simulink model "Integration2022b_May06"  (R2022b)
settings: Solver=FixedStepAuto  StartTime=0.0  StopTime=inf  RelTol=1e-3
model workspace (MAT data in the model file):
  L = 4.165
  SL_ROS_VariableLengthArrays_MaxSizes : object (value not decoded)
  finalint = 0
  firstWarning = 1
  originalScenarioChecksum = '114339432DE22364D47BB28FC96DC10C'
values from neighbouring files (symbols this model uses):
  D = cross(B-A,C-A)    [HelperCalculateEgoRefPathInfo.m]
  data =     [Part_of_MCity.mat]    (also in curvedroad_Bhanu.mat; plotWPScript.m = [data, [out.x.Data(:, :, i); out.y.Data(:, :, i)]])
  x = [Vertices(Na,1) Vertices(:,1) Vertices(Nb,1)]    [HelperCalculateEgoRefPathInfo.m]    (also in HelperConvertDSPoseToSim3D.m = actor(1).Position(1); xpts.mat = [-29.9023190589 -34.2715935353 -19.4160603154 -19.4160603154)
  y = [Vertices(Na,2) Vertices(:,2) Vertices(Nb,2)]    [HelperCalculateEgoRefPathInfo.m]    (also in HelperConvertDSPoseToSim3D.m = actor(1).Position(2); VehicleOutputFcn.m = [x(1);x(2); x(3); x(4); x(5);x(6)]; ypts.mat = [-62.3254015256 -62.9079714558 -51.8391427821 -48.6350081661)
  z = zeros(1, length(interpX))    [HelperCalculateEgoRefPathInfo.m]
undefined symbols (not defined in the file or in its folder): MinVelocity, WB
libraries: ros2lib x13, mpcsigdimcheck_private x10, robotalgslib x1, mpclib x1, drivingvehiclecontroller x1, slpidlib x1
(part 2 of 5)

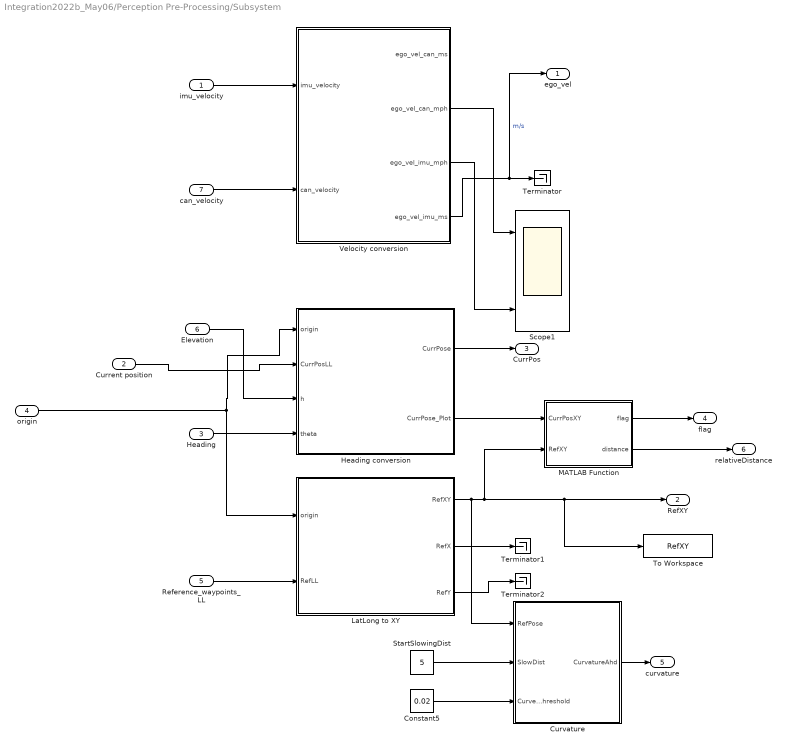
== system Integration2022b_May06/Perception Pre-Processing/Subsystem ==
  imu_velocity : Inport
  Current position : Inport  Port=2
  Heading : Inport  Port=3
  origin : Inport  Port=4
  Reference_waypoints_LL : Inport  Port=5
  Elevation : Inport  Port=6
  can_velocity : Inport  Port=7
  Constant5 : Constant  Value=0.02
  Curvature : MATLAB Function  TreatAsAtomicUnit=on
  Heading conversion : MATLAB Function  TreatAsAtomicUnit=on
  LatLong to XY : MATLAB Function  TreatAsAtomicUnit=on
  MATLAB Function : MATLAB Function  TreatAsAtomicUnit=on
  Scope1 : Scope  NumInputPorts=3
  StartSlowingDist : Constant  Value=5
  Terminator : Terminator
  Terminator1 : Terminator
  Terminator2 : Terminator
  To Workspace : ToWorkspace  VariableName=RefXY  SampleTime=-1
      settings: Save2DSignal=2-D array (concatenate along first dimension)
  Velocity conversion : MATLAB Function  TreatAsAtomicUnit=on
  ego_vel : Outport
  RefXY : Outport  Port=2
  CurrPos : Outport  Port=3
  flag : Outport  Port=4
  curvature : Outport  Port=5
  relativeDistance : Outport  Port=6
  wires:
  imu_velocity/1 -> Velocity conversion/1(imu_velocity)
  Reference_waypoints_LL/1 -> LatLong to XY/2(RefLL)
  Current position/1 -> Heading conversion/2(CurrPosLL)
  can_velocity/1 -> Velocity conversion/2(can_velocity)
  Elevation/1 -> Heading conversion/3(h)
  origin/1 -> Heading conversion/1(origin), LatLong to XY/1(origin)
  Heading/1 -> Heading conversion/4(theta)
  Velocity conversion/4(ego_vel_imu_ms) -> ego_vel/1, Terminator/1  "m/s"
  Velocity conversion/2(ego_vel_can_mph) -> Scope1/1
  Velocity conversion/3(ego_vel_imu_mph) -> Scope1/3
  Heading conversion/1(CurrPose) -> CurrPos/1
  Heading conversion/2(CurrPose_Plot) -> MATLAB Function/1(CurrPosXY)
  LatLong to XY/2(RefX) -> Terminator1/1
  LatLong to XY/3(RefY) -> Terminator2/1
  StartSlowingDist/1 -> Curvature/2(SlowDist)
  Constant5/1 -> Curvature/3(CurveMinThreshold)
  Curvature/1(CurvatureAhd) -> curvature/1
  MATLAB Function/1(flag) -> flag/1
  MATLAB Function/2(distance) -> relativeDistance/1
  LatLong to XY/1(RefXY) -> MATLAB Function/2(RefXY), To Workspace/1, RefXY/1, Curvature/1(RefPose)

== system Integration2022b_May06/Controllers/Lateral Controller/Pure Pursuit Controller1 ==
  Pose : Inport
  Waypoints : Inport  Port=2
  Pure Pursuit : robotalgslib/Pure Pursuit  DesiredLinearVelocity=5  MaxAngularVelocity=1.0  LookaheadDistance=4  TargetDirPort=on  SimulateUsing=Code generation
  Terminator6 : Terminator
  Terminator7 : Terminator
  Wheel Steering Angle Formulation : Subsystem  mask{L=2.865, ld=4}
      mask prompts: L "Bicycle length"; ld "Lookahead distance"
      mask TypeOptions L: Bicycle length/Value
      mask TypeOptions ld: Lookahead distance/Value
      mask Display:
      | image("GeometryMask.png")
      | port_label('input', 1, 'alpha')
      | port_label('output', 1, 'delta')
  delta : Outport
  wires:
  Waypoints/1 -> Pure Pursuit/2
  Wheel Steering Angle Formulation/1(Al) -> delta/1
  Pure Pursuit/3 -> Wheel Steering Angle Formulation/1(alpha)
  Pure Pursuit/2 -> Terminator7/1
  Pose/1 -> Pure Pursuit/1
  Pure Pursuit/1 -> Terminator6/1

== system Integration2022b_May06/Controllers/Longitudinal Controllers/ACC Block ==
  Relative velocity : Inport
  timeGap : Inport  Port=2
  Distance To Scene : Inport  Port=3
  defaultSpacing : Inport  Port=4
  Set velocity : Inport  Port=5
  Current Velocity : Inport  Port=6
  Adaptive Cruise Control System : Subsystem  AncestorBlock=mpclib/Automated Driving/Adaptive Cruise Control System  mask(Adaptive cruise control (ACC) system){EgoModel=tf(1,[0.5,1,0]), InitialEgoVelocity=3.6, DefaultSpacing=40, MaxVelocity=6, MinAcceleration=-3, amin_ext=off, MaxAcceleration=3, amax_ext=off, Ts=0.01, PredictionHorizon=30, ControllerBehavior=0.410, suboptimal=off, maxiter=10, datatypeopt=double, optmode=off, trackmode=off}
      mask prompts: EgoModel "MPC:adasblocks:promptACCLinearModel"; InitialEgoVelocity "MPC:adasblocks:promptACCInitialEgoVelocity"; DefaultSpacing "MPC:adasblocks:promptACCDefaultSpacing"; MaxVelocity "MPC:adasblocks:promptACCMaxVelocity"; MinAcceleration "MPC:adasblocks:promptACCMinAcceleration"; amin_ext "MPC:adasblocks:promptACCUseExternalSource"; MaxAcceleration "MPC:adasblocks:promptACCMaxAcceleration"; amax_ext "MPC:adasblocks:promptACCUseExternalSource"; Ts "MPC:adasblocks:promptACCSampleTime"; PredictionHorizon "MPC:adasblocks:promptACCPredictionSteps"; suboptimal "MPC:adasblocks:promptACCUseSubOptimal"; maxiter "MPC:adasblocks:promptACCMaxIter"; datatypeopt "MPC:adasblocks:promptACCDataType"; optmode "MPC:adasblocks:promptACCMPCOptimize"; trackmode "MPC:adasblocks:promptACCSmoothTransition"
      mask help: MPC:adasblocks:accMaskDescription
      mask init:
      | [mpcobj,MinVelocity,DataType] = accblock_MaskInitFcn(gcb,EgoModel,DefaultSpacing,MaxVelocity,...
      |                                                                     MaxAcceleration,MinAcceleration,...
      |                                                                     InitialEgoVelocity,...
      |                                                                     PredictionHorizon,Ts,maxiter,ControllerBehavior);
      mask Help: eval('mpcCSHelp(''mpcBlockACC'',''HelpBrowser'')');
      mask Callback amin_ext: adasblocks_utilUseExternal(gcb,'MinAcceleration','amin_ext');
      mask Callback amax_ext: adasblocks_utilUseExternal(gcb,'MaxAcceleration','amax_ext');
      mask Callback suboptimal: adasblocks_callbackUsesuboptimal(gcb);
      mask TypeOptions datatypeopt: double | single
      mask DialogControl DescTextVar Tooltip: MPC:adasblocks:ttipACCMaskDescription
      mask DialogControl Container18 Prompt: MPC:adasblocks:promptACCTabParameters
      mask DialogControl Container30 Prompt: MPC:adasblocks:promptACCEgoVehicle
      mask DialogControl EgoModel Prompt: Linear model from longitudinal acceleration to longitudinal velocity
      mask DialogControl EgoModel Tooltip: MPC:adasblocks:ttipACCLinearModel
      mask DialogControl InitialEgoVelocity Prompt: Initial condition for longitudinal velocity (m/s)
      mask DialogControl InitialEgoVelocity Tooltip: MPC:adasblocks:ttipACCInitialEgoVelocity
      mask DialogControl DefaultSpacing Prompt: Default spacing (m)
      mask DialogControl DefaultSpacing Tooltip: MPC:adasblocks:ttipACCDefaultSpacing
      mask DialogControl MaxVelocity Prompt: Maximum velocity (m/s)
      mask DialogControl MaxVelocity Tooltip: MPC:adasblocks:ttipACCMaxVelocity
      mask DialogControl Container22 Prompt: MPC:adasblocks:promptACCConstraints
      mask DialogControl MinAcceleration Prompt: Minimum longitudinal acceleration (m/s^2)
      mask DialogControl MinAcceleration Tooltip: MPC:adasblocks:ttipACCMaxDeceleration
      mask DialogControl amin_ext Prompt: Use external source
      mask DialogControl MaxAcceleration Prompt: Maximum longitudinal acceleration (m/s^2)
      mask DialogControl MaxAcceleration Tooltip: MPC:adasblocks:ttipACCMaxAcceleration
      mask DialogControl amax_ext Prompt: Use external source
      mask DialogControl Container9 Prompt: MPC:adasblocks:promptACCMPCSettings
      mask DialogControl Ts Prompt: Sample time (s)
      mask DialogControl Ts Tooltip: MPC:adasblocks:ttipACCSampleTime
      mask DialogControl PredictionHorizon Prompt: Prediction horizon (steps)
      mask DialogControl PredictionHorizon Tooltip: MPC:adasblocks:ttipACCPredictionSteps
      mask DialogControl Container14 Prompt: MPC:adasblocks:promptACCWeight
      mask DialogControl ControllerBehavior Tooltip: MPC:adasblocks:ttipACCWeight
      mask DialogControl SliderText Prompt: More robust            More aggressive
      mask DialogControl Container21 Prompt: MPC:adasblocks:promptACCOptionsText
      mask DialogControl Container19 Prompt: MPC:adasblocks:promptACCOptimization
      mask DialogControl suboptimal Prompt: Use suboptimal solution
      mask DialogControl suboptimal Tooltip: MPC:adasblocks:ttipACCUseSubOptimal
      mask DialogControl maxiter Prompt: Maximum iteration number
      mask DialogControl maxiter Tooltip: MPC:adasblocks:ttipACCMaxIter
      mask DialogControl datatypeopt Prompt: Data Type
      mask DialogControl datatypeopt Tooltip: MPC:adasblocks:ttipACCDataType
      mask DialogControl Container23 Prompt: MPC:adasblocks:promptACCBlockOptions
      mask DialogControl optmode Prompt: Use external signal to enable or disable optimization
      mask DialogControl optmode Tooltip: MPC:adasblocks:ttipACCMPCOptimize
      mask DialogControl trackmode Prompt: Use external control signal for bumpless transfer between ACC and other controllers
      mask DialogControl trackmode Tooltip: MPC:adasblocks:ttipACCSmoothTransition
      mask DialogControl Container25 Prompt: MPC:adasblocks:promptACCCustomizeText
      mask DialogControl Control7 Prompt: MPC:adasblocks:promptACCCreateSystemTextMore
      mask DialogControl Control3 Prompt: MPC:adasblocks:promptACCCreateSysBtn
      mask DialogControl Control3 Tooltip: MPC:adasblocks:ttipACCCreateSysBtn
      mask DialogControl Control3 Callback: accblock_callbackCreateSubsystemButton(gcb);
  MATLAB Function : MATLAB Function  TreatAsAtomicUnit=on
  acceleration : Outport
  deceleration : Outport  Port=2
  wires:
  MATLAB Function/2(deceleration) -> deceleration/1
  Relative velocity/1 -> Adaptive Cruise Control System/5(Relative velocity)
  Set velocity/1 -> Adaptive Cruise Control System/1(Set velocity)
  Adaptive Cruise Control System/1(Longitudinal acceleration) -> MATLAB Function/1(ACC_Acceleration)
  MATLAB Function/1(acceleration) -> acceleration/1
  timeGap/1 -> Adaptive Cruise Control System/2(timeGap)
  Current Velocity/1 -> Adaptive Cruise Control System/3(Longitudinal velocity)
  defaultSpacing/1 -> Adaptive Cruise Control System/6(defaultSpacing)
  Distance To Scene/1 -> Adaptive Cruise Control System/4(Relative distance)

== system Integration2022b_May06/Controllers/Longitudinal Controllers/Longitduinal Controller ==
  Distance To Scene : Inport
  safeStop : Inport  Port=2
  Slow Down Flag : Inport  Port=3
  Reference Velocity : Inport  Port=4
  Current Velocity : Inport  Port=5
  Direction : Inport  Port=6
  Reset : Inport  Port=7
  holdBrakeFlag : Inport  Port=8
  Gain : Gain  Gain=-1
  Longitudinal Controller Stanley : drivingvehiclecontroller/Longitudinal Controller Stanley  Kp=2  Ki=0.15  SampleTime=0.01  MaxAcceleration=3  MaxDeceleration=3
  MATLAB Function2 : MATLAB Function  TreatAsAtomicUnit=on
  Accel : Outport
  Decel : Outport  Port=2
  wires:
  Reference Velocity/1 -> Longitudinal Controller Stanley/1
  safeStop/1 -> MATLAB Function2/4(safeStop)
  Longitudinal Controller Stanley/1 -> MATLAB Function2/2(AccelCmd)
  Current Velocity/1 -> Longitudinal Controller Stanley/2
  Gain/1 -> MATLAB Function2/3(DecelCmd)
  Longitudinal Controller Stanley/2 -> Gain/1
  MATLAB Function2/1(Accel) -> Accel/1
  Reset/1 -> Longitudinal Controller Stanley/4
  Distance To Scene/1 -> MATLAB Function2/1(distance2Scene)
  Slow Down Flag/1 -> MATLAB Function2/5(slowDownFlag)
  Direction/1 -> Longitudinal Controller Stanley/3
  holdBrakeFlag/1 -> MATLAB Function2/6(holdBrakeFlag)
  MATLAB Function2/2(Decel) -> Decel/1

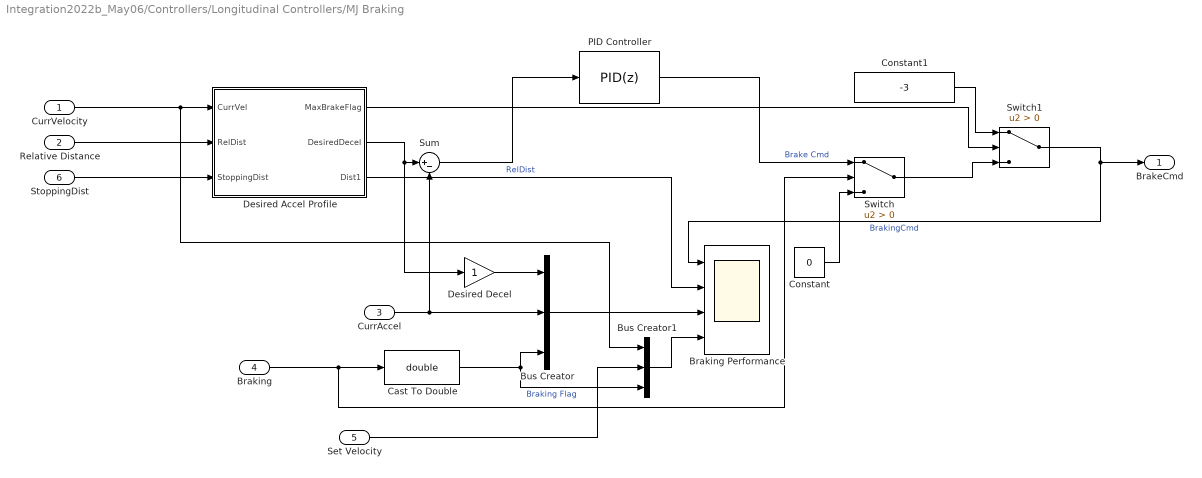
== system Integration2022b_May06/Controllers/Longitudinal Controllers/MJ Braking ==
  CurrVelocity : Inport
  Relative Distance : Inport  Port=2
  CurrAccel : Inport  Port=3
  "Braking " : Inport  Port=4
  Set Velocity : Inport  Port=5
  StoppingDist : Inport  Port=6
  Braking Performance : Scope  NumInputPorts=4
  Bus Creator : BusCreator  Inputs=3
  Bus Creator1 : BusCreator  Inputs=3
  Cast To Double : DataTypeConversion  OutDataTypeStr=double  SaturateOnIntegerOverflow=off  RndMeth=Floor
  Constant : Constant  Value=0
  Constant1 : Constant  Value=-3
  Desired Accel Profile : MATLAB Function  TreatAsAtomicUnit=on
  Desired Decel : Gain
  PID Controller : slpidlib/PID Controller  Controller=PID  Form=Parallel  TimeDomain=Discrete-time  UseExternalTs=off  SampleTime=0.01  IntegratorMethod=Forward Euler  FilterMethod=Forward Euler  ControllerParametersSource=internal  P=1.5  I=0.01  UseKiTs=off  D=0.03  N=100  UseFilter=on  TunerSelectOption=Transfer Function Based (PID Tuner App)  InitialConditionSource=internal  InitialConditionForIntegrator=0  InitialConditionForFilter=0  DifferentiatorICPrevScaledInput=0  ExternalReset=none  TrackingMode=off  Kt=1  LimitOutput=on  SatLimitsSource=internal  UpperSaturationLimit=3  LowerSaturationLimit=-3  LinearizeAsGain=on  AntiWindupMode=none  Kb=1  LimitIntegrator=off  UpperIntegratorSaturationLimit=inf  LowerIntegratorSaturationLimit=-inf  POutMin=[]  POutMax=[]  IOutMin=[]  IOutMax=[]  DOutMin=[]  DOutMax=[]  NOutMin=[]  NOutMax=[]  SumOutMin=[]  SumOutMax=[]  SaturationOutMin=[]  SaturationOutMax=[]  PParamMin=[]  PParamMax=[]  IParamMin=[]  IParamMax=[]  DParamMin=[]  DParamMax=[]  NParamMin=[]  NParamMax=[]  KbParamMin=[]  KbParamMax=[]  KtParamMin=[]  KtParamMax=[]  KbOutMin=[]  KbOutMax=[]  KtOutMin=[]  KtOutMax=[]  IntegratorOutMin=[]  IntegratorOutMax=[]  FilterOutMin=[]  FilterOutMax=[]  SumI1OutMin=[]  SumI1OutMax=[]  SumI2OutMin=[]  SumI2OutMax=[]  SumI3OutMin=[]  SumI3OutMax=[]  SumI4OutMin=[]  SumI4OutMax=[]  SumDOutMin=[]  SumDOutMax=[]  DifferentiatorOutMin=[]  DifferentiatorOutMax=[]  FilterDiffOutCoefMin=[]  FilterDiffOutCoefMax=[]  ReciprocalOutMin=[]  ReciprocalOutMax=[]  SumDenOutMin=[]  SumDenOutMax=[]  SumNumOutMin=[]  SumNumOutMax=[]  DivideOutMin=[]  DivideOutMax=[]  UdiffTsProdOutMin=[]  UdiffTsProdOutMax=[]  NTsProdOutMin=[]  NTsProdOutMax=[]  UintegralTsProdOutMin=[]  UintegralTsProdOutMax=[]  UngainTsProdOutMin=[]  UngainTsProdOutMax=[]  IntegratorContinuousStateAttributes=''  IntegratorStateMustResolveToSignalObject=off  IntegratorRTWStateStorageClass=Auto  FilterContinuousStateAttributes=''  FilterStateMustResolveToSignalObject=off  FilterRTWStateStorageClass=Auto  ParallelPVariant=InternalParameters  IdealPVariant=Disabled  IVariant=InternalParameters  DVariant=InternalParameters  IntegratorVariant=Discrete  SatVariant=Enabled  AWVariant=Passthrough  PCopyVariant=Disabled  TRVariant=Disabled  FdbkBlocksVariant=Forward  IdealPFdbkVariant=Disabled  SatFdbkVariant=Disabled  DerivativeFilterVariant=ForwardEulerFilter  NVariant=InternalParameters  NCopyVariant=Disabled  FilterICVariant=InternalICsFilter  IntegratorICVariant=InternalICs  ExternalResetVariant=Disabled  TRSumVariant=Passthrough  SumFdbkVariant=Disabled  SumVariant=Sum_PID  TsampFilterVariant=InternalTs  TsampNgainVariant=Passthrough  TsampIntegralVariant=Disabled_SignalSpec  ExternalSaturationOutDataTypeStr=Inherit: Same as second input
  Sum : Sum  Inputs=|+-
  Switch : Switch  Criteria=u2 > Threshold  SaturateOnIntegerOverflow=off  InputSameDT=off
  Switch1 : Switch  Criteria=u2 > Threshold  SaturateOnIntegerOverflow=off  InputSameDT=off
  BrakeCmd : Outport
  wires:
  StoppingDist/1 -> Desired Accel Profile/3(StoppingDist)
  Set Velocity/1 -> Bus Creator1/2
  Bus Creator1/1 -> Braking Performance/4
  Desired Accel Profile/1(MaxBrakeFlag) -> Switch1/2
  Constant1/1 -> Switch1/1
  Switch/1 -> Switch1/3
  Desired Accel Profile/3(Dist1) -> Braking Performance/2  "RelDist"
  Cast To Double/1 -> Bus Creator/3, Bus Creator1/3  "Braking Flag"
  Bus Creator/1 -> Braking Performance/3
  Switch1/1 -> Braking Performance/1, BrakeCmd/1  "BrakingCmd"
  Constant/1 -> Switch/3
  Desired Decel/1 -> Bus Creator/1
  CurrAccel/1 -> Sum/2, Bus Creator/2
  PID Controller/1 -> Switch/1  "Brake Cmd"
  "Braking "/1 -> Switch/2, Cast To Double/1
  Desired Accel Profile/2(DesiredDecel) -> Desired Decel/1, Sum/1
  Sum/1 -> PID Controller/1
  CurrVelocity/1 -> Bus Creator1/1, Desired Accel Profile/1(CurrVel)
  Relative Distance/1 -> Desired Accel Profile/2(RelDist)

== system Integration2022b_May06/Controllers/Longitudinal Controllers/Profile Generator ==
  desiredVelocity : Inport
  safeStopDistance : Inport  Port=2
  Distance To Scene : Inport  Port=3
  Slow Down Flag : Inport  Port=4
  Current Velocity : Inport  Port=5
  Memory2 : Memory  InheritSampleTime=on
  Memory3 : Memory  InitialCondition=zeros(6,1)  InheritSampleTime=on
  Profile Generator : MATLAB Function  TreatAsAtomicUnit=on
  Reference Velocity : Outport
  wires:
  Distance To Scene/1 -> Profile Generator/1(distanceToScene)
  Profile Generator/3(a_coeff) -> Memory3/1
  safeStopDistance/1 -> Profile Generator/3(safeStopDistance)
  Profile Generator/2(X_f) -> Memory2/1
  Current Velocity/1 -> Profile Generator/4(CurrVel)
  Memory2/1 -> Profile Generator/6("X_f ")
  desiredVelocity/1 -> Profile Generator/5(desiredVelocity)
  Memory3/1 -> Profile Generator/7("a_coeff ")
  Profile Generator/1(referenceVelocity) -> Reference Velocity/1  "Reference Velocity"
  Slow Down Flag/1 -> Profile Generator/2(slowDownFlag)

== system Integration2022b_May06/Controllers/Lateral Controller/Pure Pursuit Controller1/Wheel Steering Angle Formulation ==
  alpha : Inport
  Bicycle length : Constant  Value=L
  Constant : Constant  Value=2
  Divide : Product  Inputs=*/
  Lookahead distance : Constant  Value=ld
  Product : Product
  Product1 : Product
  Sine Wave : Sin  TimeSource=Use external signal  SampleTime=0
  Trigonometric Function : Trigonometry  Operator=atan
  Al : Outport
  wires:
  Sine Wave/1 -> Product1/2
  Bicycle length/1 -> Product/2
  Constant/1 -> Product/1
  Product1/1 -> Divide/1
  Product/1 -> Product1/1
  Divide/1 -> Trigonometric Function/1
  Trigonometric Function/1 -> Al/1
  alpha/1 -> Sine Wave/1
  Lookahead distance/1 -> Divide/2

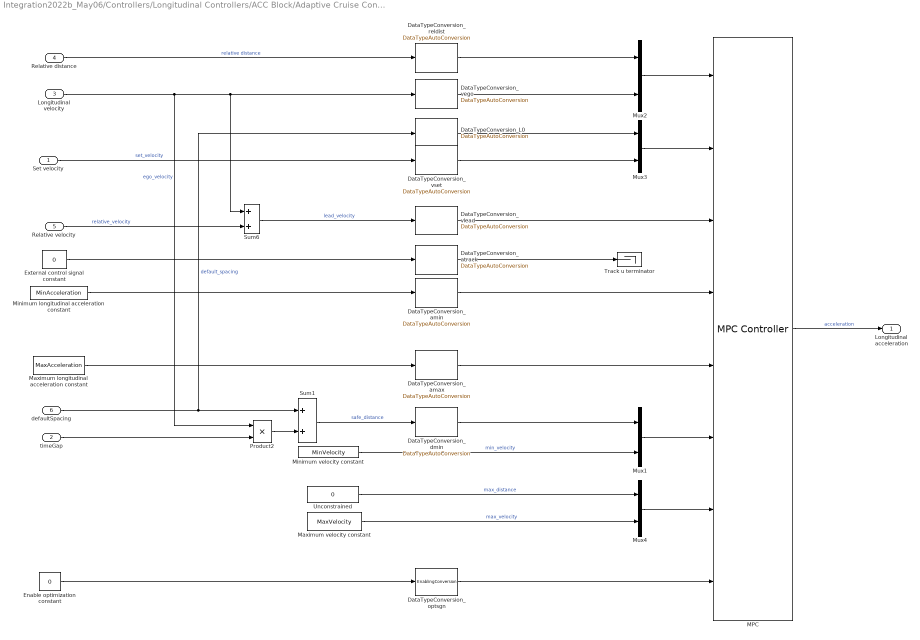
== system Integration2022b_May06/Controllers/Longitudinal Controllers/ACC Block/Adaptive Cruise Control System ==
  Set velocity : Inport
  timeGap : Inport  Port=2
  Longitudinal velocity : Inport  Port=3
  Relative distance : Inport  Port=4
  Relative velocity : Inport  Port=5
  defaultSpacing : Inport  Port=6
  DataTypeConversion_L0 : mpcsigdimcheck_private/DataTypeAutoConversion  datatypestr=DataType
  DataTypeConversion_amax : mpcsigdimcheck_private/DataTypeAutoConversion  datatypestr=DataType
  DataTypeConversion_amin : mpcsigdimcheck_private/DataTypeAutoConversion  datatypestr=DataType
  DataTypeConversion_atrack : mpcsigdimcheck_private/DataTypeAutoConversion  datatypestr=DataType
  DataTypeConversion_dmin : mpcsigdimcheck_private/DataTypeAutoConversion  datatypestr=DataType
  DataTypeConversion_optsgn : mpcsigdimcheck_private/EnablingConversion  SystemSampleTime=-1  VariantActivationTime=update diagram  Latency=0  AutoFrameSizeCalculation=off
  DataTypeConversion_reldist : mpcsigdimcheck_private/DataTypeAutoConversion  datatypestr=DataType
  DataTypeConversion_vego : mpcsigdimcheck_private/DataTypeAutoConversion  datatypestr=DataType
  DataTypeConversion_vlead : mpcsigdimcheck_private/DataTypeAutoConversion  datatypestr=DataType
  DataTypeConversion_vset : mpcsigdimcheck_private/DataTypeAutoConversion  datatypestr=DataType
  Enable optimization constant : Constant  Value=0
  External control signal constant : Constant  Value=0  OutDataTypeStr=double
  MPC : mpclib/MPC Controller  SCDEnableBlockLinearizationSpecification=on  mpcobj=mpcobj  is_multiple=0  enable_value=0  return_u0=off  updateMPCinCallerWorkspace=off  md_inport=on  mv_inport=off  uref_inport=off  return_cost=off  return_mvseq=off  return_qpstatus=off  return_xseq=off  return_state=off  return_ovseq=off  state_inport=off  umin_inport=on  umax_inport=on  ymin_inport=on  ymax_inport=on  cc_inport=off  ywt_inport=off  uwt_inport=off  duwt_inport=off  rhoeps_inport=off  pm_inport=off  MaximumP=10  HorizonChoice=FixedHorizon  n_ts=0.01  n_p=30  n_mv=1  n_md=1  n_ud=0  n_mo=2  n_uo=0  BlockDataType=double  SampleTimeInherited=off  switch_inport=on
      settings: LibrarySourceBlock=mpclib/Automated Driving/Adaptive Cruise Control System/MPC
  Maximum longitudinal acceleration constant : Constant  Value=MaxAcceleration
  Maximum velocity constant : Constant  Value=MaxVelocity  OutDataTypeStr=DataType
  Minimum longitudinal acceleration constant : Constant  Value=MinAcceleration
  Minimum velocity constant : Constant  Value=MinVelocity  OutDataTypeStr=DataType
  Mux{1..4} (4 alike) : Mux  Inputs=[1 1]
  Product2 : Product
  Sum1 : Sum
  Sum6 : Sum
  Track u terminator : Terminator
  Unconstrained : Constant  Value=0  OutDataTypeStr=DataType
  Longitudinal acceleration : Outport  PortDimensions=1  VectorParamsAs1DForOutWhenUnconnected=off
  wires:
  Sum6/1 -> DataTypeConversion_vlead/1  "lead_velocity"
  defaultSpacing/1 -> DataTypeConversion_L0/1, Sum1/1  "default_spacing"
  Mux2/1 -> MPC/1
  Mux3/1 -> MPC/2
  Longitudinal velocity/1 -> Product2/1, DataTypeConversion_vego/1, Sum6/1  "ego_velocity"
  Relative distance/1 -> DataTypeConversion_reldist/1  "relative distance"
  Relative velocity/1 -> Sum6/2  "relative_velocity"
  MPC/1 -> Longitudinal acceleration/1  "acceleration"
  Product2/1 -> Sum1/2
  Minimum velocity constant/1 -> Mux1/2  "min_velocity"
  Sum1/1 -> DataTypeConversion_dmin/1  "safe_distance"
  Mux1/1 -> MPC/6
  DataTypeConversion_amax/1 -> MPC/5
  DataTypeConversion_amin/1 -> MPC/4
  DataTypeConversion_dmin/1 -> Mux1/1
  DataTypeConversion_vlead/1 -> MPC/3
  DataTypeConversion_L0/1 -> Mux3/1
  DataTypeConversion_vset/1 -> Mux3/2
  DataTypeConversion_reldist/1 -> Mux2/1
  DataTypeConversion_vego/1 -> Mux2/2
  timeGap/1 -> Product2/2
  Set velocity/1 -> DataTypeConversion_vset/1  "set_velocity"
  Minimum longitudinal acceleration constant/1 -> DataTypeConversion_amin/1
  Maximum longitudinal acceleration constant/1 -> DataTypeConversion_amax/1
  Mux4/1 -> MPC/7
  Maximum velocity constant/1 -> Mux4/2  "max_velocity"
  Unconstrained/1 -> Mux4/1  "max_distance"
  Enable optimization constant/1 -> DataTypeConversion_optsgn/1
  DataTypeConversion_optsgn/1 -> MPC/8
  External control signal constant/1 -> DataTypeConversion_atrack/1
  DataTypeConversion_atrack/1 -> Track u terminator/1

== matlab function Integration2022b_May06/Perception Pre-Processing/Subsystem/Velocity conversion ==
  data: ego_vel_can_ms output; imu_velocity input; can_velocity input; ego_vel_can_mph output; ego_vel_imu_mph output; ego_vel_imu_ms output
function [ego_vel_can_ms, ego_vel_can_mph, ego_vel_imu_mph, ego_vel_imu_ms] = fcn(imu_velocity, can_velocity)


ego_vel_can_ms = double(can_velocity(1)) * 0.27778;  %kmh to m/s
ego_vel_can_mph = ego_vel_can_ms * 2.237; %m/s to mph

ego_vel_imu_ms = double(imu_velocity(1));  % m/s
ego_vel_imu_mph = ego_vel_imu_ms * 2.237; %m/s 


end

== matlab function Integration2022b_May06/Perception Pre-Processing/Orientation (from GPS) ==
  data: ego_vel output; CurrentPos output; heading output; imuData input; gpsData input
function [ego_vel, CurrentPos, heading] = fcn(imuData, gpsData)
imu = double(imuData(1:2));
gps = double(gpsData(1:2));

lat = (gps(1));
long = (gps(2));

heading = (imu(1));
ego_vel = (imu(2));

CurrentPos=[lat long];

end

== matlab function Integration2022b_May06/Perception Pre-Processing/Lane markings ==
  data: u input; y output
function y = fcn(u)
if any(u, "all")
    u1 = u(1:315);
    y = double(reshape(u1, 63, 5));
else
   y = double(-1*ones(63, 5));
end

== matlab function Integration2022b_May06/Stop Controller/Brake Safety ==
  data: deceleration input; actualDeceleration output; flag input; velocity input; steering input
function actualDeceleration = fcn(deceleration, flag, velocity, steering)

    if abs(velocity) <= 0.2 && flag == 1 && abs(steering) <= 22.5
        actualDeceleration = 0;
    else
        actualDeceleration = deceleration;
    end
end

== matlab function Integration2022b_May06/Stop Controller/MATLAB Function5 ==
  data: acceleration input; stopSimFlag output; braking input; steering input; velocity input; flag input
function stopSimFlag = fcn(acceleration, braking, steering, velocity, flag)
    
    if abs(acceleration) <= 0.4 && abs(braking) <= 0.4 && abs(steering) <= 22.5 && abs(velocity) <= 0.2 && flag == 1
        stopSimFlag = 1;
    else
        stopSimFlag = 0;
    end
end

== matlab function Integration2022b_May06/Stop Controller/Steer Safety ==
  data: steering input; actualSteeringCommand output; flag input
function actualSteeringCommand = fcn(steering, flag)

    if flag == 1
        actualSteeringCommand = 0;
    else
        actualSteeringCommand = steering;
    end
end

== matlab function Integration2022b_May06/Behavioural Planner/MATLAB Function1 ==
  data: EgoLength input; TransDist output; IntDist input
function TransDist = IntersectionClearanceDist(EgoLength,IntDist)

TransDist = IntDist + EgoLength;

== matlab function Integration2022b_May06/Perception Pre-Processing/Limit lines ==
  data: u input; y output; origin input
function y = fcn(u, origin)
if any(u, "all")
    u1 = u(1:378);
    y = double(reshape(u1, 6, 63))';
    height = ones(63, 1) * 229;
    limitLineLL = [y(:, 5), y(:, 6), height];
    limitLineXY =  lla2enu(limitLineLL, origin, 'ellipsoid');                   % Traffic Sign Lat-Long to XY Coordinate Conversion
    y(:, 5) = limitLineXY(:, 1);
    y(:, 6) = limitLineXY(:, 2);
else
   y = double(-1*ones(6, 63))';
end
end

== stateflow chart Integration2022b_May06/Behavioural Planner/Behavioural Planner/Collision Avoidance ==
  state Stop
    en:
    Brake = 1;
  state Start
    en:
    Stuck = 0;
    ACC = 0;
    LaneChangeCmd = 0;
    %VelCmd = CurrentVelCmd;
  state Follow
    en:
    ACC = 1;
    Brake = 0;
  state LaneChange
    en:
    LaneChangeCmd = 1;
    ACC=0;
  Stop -> Follow : [EgoSpeed<0.1]
  Follow -> Stop [order 4] : [D2O < 10 && EgoSpeed > 2]
  (default) -> Start
  Follow -> LaneChange [order 2] : [LC_ACC==1]
  Start -> Follow : [ObjAhead == 1 && D2O < 20]
  Follow -> Start [order 3] : [ObjAhead == 0]
  LaneChange -> Start : [LaneChanged == 1]
  Follow -> Follow [order 1] : [(EgoSpeed <= MinSpeed) && after(WaitTime,sec)]{Stuck = 1;}
  data: Stuck local; ACC output; WaitTime input; ObjAhead input; MinSpeed input; LaneAvailable input; EgoSpeed input; LaneChanged input; LC_ACC input; LaneChangeCmd output; Brake output; D2O input

== matlab function Integration2022b_May06/LaneChange_BehavioralModel ==
  data: A input; RLChange output; LLChange output; LChange output; egovel input; objahead input; relvel input; objdist input; RoadSpeed input; LLMarking input; RLMarking input; egoLane input; numLane input
function [RLChange, LLChange, LChange] = fcn(A, egovel, objahead, relvel, objdist, RoadSpeed, LLMarking, RLMarking, egoLane, numLane)  % the code is written for only straight roads
RLChange = 0;  %% Flag to facilitate right lane change
LLChange = 0;  %% Flag to facilitate left lane change
LChange = 0; %% Flag to notify a lane change

%%
lanechangereq = 0;
r_c = 20; %range considered to MIOs
t_min =  2; 
sameLaneObjDist = 20;
sa = size(A);
dist = zeros(sa);
ttc = zeros(sa);
flagLL = 0;
flagRL = 0;
LLChange_flag = zeros(1, 2); %% used to see which cases give left lane change possible. 
RLChange_flag = zeros(1, 2); %% used to see which cases give right lane change possible. 
%%


if objahead && relvel < 0 && objdist < sameLaneObjDist %%&& egovel < (RoadSpeed+5)
    lanechangereq = 1;
end


for i = 1:sa(1)
    dist(i) = A(i, 4); %only accounting for the longitudinal distance of the object from the car
    ttc(i) = dist(i)/abs(A(i, 5));
end
%% version -1 
% 
% % for i = 1:sa(1)
% %     if lanechangereq
% %         if A(i,6) == 5 && dist(i) > r_c && ttc(i) > t_min && RLMarking(1) ~= 2 && (RLMarking(2) )
% %             RLChange = 1;
% %         end
% %     end
% % end
% 
% for i = 1:sa(1)
%     if lanechangereq
%         if A(i,6) == 5
%             flagRL = 1; %% right lane exists
%             if dist(i) > r_c && ttc(i) > t_min  %% an object on the right lane detected and object is far enough to make lane change 
%                 RLChange = 1;
%             else
%                 flagRL = 2;
%             end
%         elseif A(i,6) == 4 
%             flagLL = 1; %%left lane exists
%             if dist(i) > r_c && ttc(i) > t_min  %% an object on the left lane detected and object is far enough to make lane change 
%                 LLChange = 1;
%             else
%                 flagLL = 2;
%             end
%         end
% 
%         if flagRL == 0 && RLMarking(1) == 1 && (RLMarking(2) == 2 || RLMarking(2) == 3 || RLMarking(2) == 4)
%             RLChange = 1;
%         end
%         if flagLL == 0 && LLMarking(1) == 1 && (LLMarking(2) == 2 || LLMarking(2) == 3 || LLMarking(2) == 4)
%             LLChange = 1;
%         end
%     end
% end
% 
% 
% if (RLChange || LLChange)
%     LChange = 1;
% end


%%version - 2  %% I have information about the number of lanes and the
%%exact lane which the ego vehicle is in. (Number of lanes includes all
%%lanes in both directions. -> have this information but did not use it
%%yet. couldbe used for future versions of the code. 

    for i = 1:sa(1)
        if lanechangereq
            if A(i,6) == 4 && dist(i) > r_c && ttc(i) > t_min %% there is an object in the left lane and it far enough to make a lane change
                LLChange_flag(1) = 1;
                flagLL = 1; %% left lane detection done
            end
            if A(i, 6) == 5 && dist(i) > r_c && ttc(i) > t_min %% there is an object in the right lane and it far enough to make a lane change
                RLChange_flag(1) = 1;
                flagRL = 1; %% right lane detection done
            end
            if ~flagLL && LLMarking(1) == 1 && (LLMarking(2) == 2 || LLMarking(2) == 3 || LLMarking(2) == 4) %% no object was found on the left lane but it is legal to make a left lane change (white dashed left line)
                LLChange_flag(2) = 1;
            end
            if ~flagRL && RLMarking(1) == 1 && (RLMarking(2) == 2 || RLMarking(2) == 3 || RLMarking(2) == 4) %% no object was found on the right lane but it is legal to make a right lane change (white dashed right line)
                RLChange_flag(2) = 1;
            end
        end
    end

% LLChange = LLChange_flag(1) || LLChange_flag(2);
% RLChange = RLChange_flag(1) || RLChange_flag(2) && ~LLChange; %% giving higher priority to left lane change. if Left lane change is possible then right lane change wont be executed.

if LLChange_flag(1) || LLChange_flag(2)
    LLChange = 1;
end

if ~LLChange && RLChange_flag(1) || RLChange_flag(2)
    RLChange = 1;
end
if RLChange || LLChange
    LChange = 1;
end

== stateflow chart Integration2022b_May06/Behavioural Planner/Subsystem/Chart1 ==
  settings: updateMethod=DISCRETE  sampleTime=Ts
  state Stationary
    en,du:
    VelCmd = 0;
    CurrentVelCmd = VelCmd;
    Navi = 0;
    Trans = 0;
    StopSim = 0;
    Tgap = 1;
    HoldBrake = 1;
    Braking = 0;
  state Navigation
    state RailCrossing
      state Stop
        en:
        VelCmd = 0;
        Braking = 1;
        CurrentVelCmd = VelCmd;
      state Approaching
        en:
        Braking = 1;
        Tgap = 0;
        Trans = 0;
      state Transition
        en:
        Tgap = 1;
        Trans = 1;
        Braking = 0;
        VelCmd = SceneSpeed;
        CurrentVelCmd = VelCmd;
      state ExitScene
        en:
        ExitFlag = 1;
      (default) -> Navigation.RailCrossing.Approaching
      Navigation.RailCrossing.Approaching -> Navigation.RailCrossing.Stop [order 1] : [D2S <= 6 && (RRCross == 1 || ObjectDist <= TransDist)]
      Navigation.RailCrossing.Transition -> Navigation.RailCrossing.Approaching [order 2] : [ObjectDist <= TransDist]
      Navigation.RailCrossing.Approaching -> Navigation.RailCrossing.Transition [order 3] : [RRCross == 0 && ObjectDist > TransDist && D2S <= 6]
      Navigation.RailCrossing.Stop -> Navigation.RailCrossing.Transition : [RRCross == 0 && ObjectDist > TransDist]
      Navigation.RailCrossing.Approaching -> Navigation.RailCrossing.ExitScene [order 2] : [SceneID ~= 10]
      Navigation.RailCrossing.Transition -> Navigation.RailCrossing.ExitScene [order 1] : [SceneID == 0]
    state RoundAbout
      state Approaching
        en:
        Braking = 1;
        Trans = 0;
        Tgap = 0;
      state Stop
        en:
        VelCmd = 0;
        Braking = 1;
        CurrentVelCmd = VelCmd;
      state ExitScene
        en:
        ExitFlag = 1;
      state Transition
        en:
        Tgap = 1;
        Trans = 1;
        Braking = 0;
        VelCmd = SceneSpeed;
        CurrentVelCmd = VelCmd;
      (default) -> Navigation.RoundAbout.Approaching
      Navigation.RoundAbout.Approaching -> Navigation.RoundAbout.Stop [order 1] : [D2S <= 6]
      Navigation.RoundAbout.Stop -> Navigation.RoundAbout.Transition : [Clear2Go == 1]
      Navigation.RoundAbout.Approaching -> Navigation.RoundAbout.ExitScene [order 2] : [SceneID ~= 9]
      Navigation.RoundAbout.Transition -> Navigation.RoundAbout.ExitScene : [SceneID == 0]
    state DestCheck
      en,du:
      % dest reached?
      (default) -> (junction 47)
      (junction 47) -> (junction 48) [order 1] : [D2D < 2]
      (junction 47) -> (junction 49) [order 2] : {DestReached = 0;}
      (junction 48) -> (junction 50) : {DestReached = 1;}
      (junction 50) -> (junction 49) : {StopSim = 1;}
      (junction 49) -> (junction 51)
    state TrafficLight [commented out]
      note: Yellow light duration is 1s
      state Stop [commented out]
        en:
        Braking = 1;
        VelCmd = 0;
        CurrentVelCmd = VelCmd;
      state Approaching [commented out]
        en:
        Tgap = 0;
        Trans = 0;
        T2S = 0;
        %if TLstate(1,4) == 1
        Braking = 1;
        %else
        % ACC = 0;
        %end
      state DecisionOnYellow [commented out]
        en:
        T2S = D2S/EgoSpeed;
      state Transition [commented out]
        en:
        Trans = 1;
        Braking = 0;
        Tgap = 1;
        VelCmd = SceneSpeed;
        CurrentVelCmd = VelCmd;
      state ExitScene [commented out]
        en:
        ExitFlag = 1;
      DecisionOnYellow -> Navigation.TrafficLight.Approaching [commented out] : [T2S > 1.2]
      (default) -> Navigation.TrafficLight.Approaching [commented out]
      Navigation.TrafficLight.Approaching -> Navigation.TrafficLight.Stop [commented out] : [D2S <= 6]
      Navigation.TrafficLight.Stop -> Navigation.TrafficLight.Transition [commented out] : [TLstate(1,4) == 3 && ObjectDist > TransDist]
      Navigation.TrafficLight.Transition -> Navigation.TrafficLight.Approaching [commented out] : [TLstate(1,4) == 1  || ObjectDist < TransDist]
      Navigation.TrafficLight.Approaching -> Navigation.TrafficLight.Transition [commented out] : [TLstate(1,4) == 3 && ObjectDist > TransDist]
      Navigation.TrafficLight.Approaching -> Navigation.TrafficLight.ExitScene [commented out] : [SceneID ~= 8]
      Navigation.TrafficLight.Transition -> DecisionOnYellow [commented out] : [TLstate(1,4) == 2]
      DecisionOnYellow -> Navigation.TrafficLight.Transition [commented out] : [T2S <= 1.2]
      Navigation.TrafficLight.Transition -> Navigation.TrafficLight.ExitScene [commented out] : [SceneID == 0]
    state Drive
      en :
      HoldBrake = 0;
      VelCmd = RoadSpeed;
      CurrentVelCmd = VelCmd;
      ExitFlag = 0;
    state Go
      en:
      VelCmd = RoadSpeed;
      CurrentVelCmd = VelCmd;
      Trans = 0;
      ExitFlag = 0;
      Braking = 0;
      HoldBrake = 1;
    state StopSign
      state StoptSign4way
        state CheckInt
          du:
          % stopped?
          % ss priority?
        state CheckSS
          % stopped?
          % ss priority?
        state Transition
          en:
          % stay here while trans?!
          % while ~crossedLimitLine of TargetLane
          Trans = 1;
          Braking = 0;
          Tgap = 1;
          VelCmd = SceneSpeed;
          CurrentVelCmd = VelCmd;
        state ExitScene
          en:
          ExitFlag = 1;
        (default) -> Navigation.StopSign.StoptSign4way.CheckSS
        Navigation.StopSign.StoptSign4way.CheckSS -> Navigation.StopSign.StoptSign4way.CheckInt : [EgoSpeed < VelStop]
        Navigation.StopSign.StoptSign4way.CheckInt -> Navigation.StopSign.StoptSign4way.Transition : [egoSSPriority == 1 && Clear2Go == 1]
        Navigation.StopSign.StoptSign4way.Transition -> Navigation.StopSign.StoptSign4way.ExitScene : [SceneID == 0 && after(2,sec)]
      state SStype
        state Approaching
          en:
          %VelCmd = ApproachingSpeed;
          Braking = 1;
          Trans = 0;
          Tgap = 0;
        state Stop
          en:
          VelCmd = 0;
          Braking = 1;
          CurrentVelCmd = VelCmd;
        Navigation.StopSign.SStype.Stop -> 410 [order 1] : [numSS == 4]
        (default) -> Navigation.StopSign.SStype.Approaching
        Navigation.StopSign.SStype.Approaching -> Navigation.StopSign.SStype.Stop : [D2S <= 15]
        Navigation.StopSign.SStype.Stop -> 414 [order 2] : [numSS == 2]
      state StopSign2way
        state CheckInt
          en:
          VelCmd = 0;
          HoldBrake = 1;
          CurrentVelCmd = VelCmd;
        state CheckSS
          % stopped?
          % ss priority?
        state Transition1
          en:
          % stay here while trans?!
          % while ~crossedLimitLine of TargetLane
          Trans = 1;
          Braking = 0;
          HoldBrake = 0;
          Tgap = 1;
          VelCmd = SceneSpeed;
          CurrentVelCmd = VelCmd;
        state ExitScene1
          en:
          ExitFlag = 1;
        (default) -> Navigation.StopSign.StopSign2way.CheckSS
        Navigation.StopSign.StopSign2way.CheckSS -> Navigation.StopSign.StopSign2way.CheckInt : [EgoSpeed < VelStop]
        Navigation.StopSign.StopSign2way.CheckInt -> Transition1 : [egoSSPriority == 1 && ToAClearance == 1 && after(1,sec)]
        Transition1 -> Navigation.StopSign.StopSign2way.CheckInt [order 2] : [ToAClearance == 0]
        Transition1 -> ExitScene1 [order 1] : [SceneID == 0 && egoExit == 1]
      (default) -> SStype
      416 -> StoptSign4way
      411 -> StopSign2way
    Go -> RailCrossing [order 2] : [SceneID == 10]
    Drive -> RailCrossing [order 1] : [SceneID == 10]
    RailCrossing -> Go : [ExitFlag == 1]
    Go -> RoundAbout [order 3] : [SceneID == 9]
    Drive -> RoundAbout [order 2] : [SceneID == 9]
    RoundAbout -> Go : [ExitFlag == 1]
    (default) -> DestCheck
    Drive -> TrafficLight [commented out] : [SceneID == 8]
    DestCheck -> Drive : [DestReached == 0]
    Go -> TrafficLight [commented out] : [SceneID == 8]
    Drive -> DestCheck [order 4] : [D2D < 2]
    TrafficLight -> Go [commented out] : [ExitFlag == 1]
    Drive -> StopSign [order 3] : [SceneID == 7]
    Go -> DestCheck [order 1] : [SceneID == 0]
    StopSign -> Go : [ExitFlag == 1]
    Go -> StopSign [order 4] : [SceneID == 7]
  (default) -> Stationary
  Stationary -> Navigation : [Navigate == 1]
  Navigation -> Stationary : [Navigate == 0 || DestReached == 1]
  data: TLstate input; numSS input; egoExit input; ToAClearance input; TransDist input; ApproachingSpeed input; EgoSpeed input; ObjectDist input; SceneSpeed input; SDist input; RRCross input; D2S input; DestReached local; Navigate input; ExitFlag local; D2D input; Clear2Go input; RoadSpeed input; CurrentVelCmd local; Navi local; VelCmd output; HoldBrake output; SceneID input; Tgap output; Trans output; StopSim output; Braking output; T2S local; VelStop input; egoSSPriority input

== stateflow chart Integration2022b_May06/Behavioural Planner/Behavioural Planner/Emergency Stop ==
  state EmergencyCheck
    en:
    EStop = 0;
  state Pullover
    en:
    EStop=1;
  state Stop
    en:
    EStop=2;
  Pullover -> EmergencyCheck : [TechFailure == 0]
  (default) -> EmergencyCheck
  EmergencyCheck -> Pullover [order 1] : [TechFailure == 1]
  EmergencyCheck -> Stop [order 2] : [D2O<=1]
  Stop -> EmergencyCheck : [D2O > 2]
  data: D2O input; TechFailure input; EStop output

== matlab function Integration2022b_May06/Behavioural Planner/Subsystem/StopSignPriority ==
  settings: updateMethod=DISCRETE
  data: ToAClearance output; SDist input; distanceToScene input; objectTracks input; sceneId input; mostImportantObjectPose input; egoSSPriority output; egoPose input; egoSpeed input; numSS output; WB input; d output; flag input; flag output; midPoint input; midPoint output; egoExit output; egoEnter input; egoEnter output; process input; process output
function [ToAClearance, egoSSPriority, numSS, d, flag, midPoint, egoExit, egoEnter, process]  = StopSignPriority(SDist, distanceToScene, objectTracks, sceneId, mostImportantObjectPose, egoPose, egoSpeed, WB, flag, midPoint, egoEnter, process)
% calculate covariance matrix outside, input to this block is modified with final, unique detections
% egoPose = [-egoPose(2) egoPose(1) 90+egoPose(3)];

persistent SSPriority C1x C2y C3x C4y


% find number of signs (until we reach 0 valued columns)

numSS = 0;
if any(mostImportantObjectPose(:,1))
    numSS = 1;
end
end

% find number of cars

numCars = 0;
for j = 1:length(objectTracks(1,:))
    if any(objectTracks(:,j))
        numCars = numCars + 1;
    end
end


egoSSPriority = 1;
ToAClearance = 1;
ActorHeading = zeros(4,1);
actorExitang = zeros(4,1);
amax = 3;
ta = SceneSpeed/amax;
dd = 0.5*amax*(ta^2);
tcs = (19-dd)/SceneSpeed;
tt = ta + tcs;
tsafe = 1; % Adjusted for other conditions (e,g. weather, road condition ...)
ToAThreshold = tt + tsafe;
% tempPriority = zeros(numCars+1,1);
d = zeros(10, 5); % distance, velocity, time, location (wrt ego), exit (leaving ints)
Objang = zeros(10, 1);
% priorityTable = zeros(numCars+1, 5);
egoExitang = egoPose(3) - atan2d(midPoint(2)-egoPose(2),midPoint(1)-egoPose(1)); % 0 deg = straight , + = right
egoExitdist = sqrt((midPoint(2)-egoPose(2))^2+(midPoint(1)-egoPose(1))^2);

if abs(egoExitang) >= 135 && egoExitdist >= 10
    d(1,5) = 1; % ego left the ints
    egoEnter = 0;
    flag = 0;
elseif abs(egoExitang) >= 135 && egoExitdist <= 20 && egoExitdist >= 10
    d(1,5) = 1;
end

egoExit = d(1,5);


if (distanceToScene <= SDist || egoEnter == 1) && process % && egoExitdist >= 12

    % [~, index] = min(abs(mostImportantObjectPose(1,:)'));
    if numSS > 0

        Vmd = [-egoSpeed*sind(egoPose(3)), egoSpeed*cosd(egoPose(3))];
        rot = [cosd(egoPose(3)) -sind(egoPose(3)); sind(egoPose(3)) cosd(egoPose(3))];
        

        % intersection region
        if flag == 0
            C1x = min(mostImportantObjectPose(1, 1:numSS)) - (WB + 3);
            C2y = min(mostImportantObjectPose(3, 1:numSS)) - (WB + 3);
            C3x = max(mostImportantObjectPose(1, 1:numSS)) + (WB + 3);
            C4y = max(mostImportantObjectPose(3, 1:numSS)) + (WB + 3);
            C1 = rot*[C1x; C2y] + egoPose(1:2)';
            C2 = rot*[C3x; C4y] + egoPose(1:2)';
            midPoint = (C1+C2)./2;
            
            % C1x = min(mostImportantObjectPose(1, 1:numSS)) - (WB + 3);
            % C2y = min(mostImportantObjectPose(3, 1:numSS)) - (WB + 3);
            % C3x = max(mostImportantObjectPose(1, 1:numSS)) + (WB + 3);
            % C4y = max(mostImportantObjectPose(3, 1:numSS)) + (WB + 3);
            % midpoint = [2*egoPose(1)-C4y-C2y; 2*egoPose(2)+C1x+C3x]./2;
        %   scatter(-mostImportantObjectPose(3,:)+egoPose(1),mostImportantObjectPose(1,:)+egoPose(2),'blue','filled')   
            % scatter(midpoint(1), midpoint(2), 'blue', 'filled')
            % rectangle('Position',[egoPose(1)-C4y egoPose(2)+C1x abs(C4y-C2y) abs(C3x-C1x)])
            flag = C1x;
        end

        midpoint_ego = rot'*(midPoint - egoPose(1:2)');
        
        % loop through num of cars (j)
    
        d(1,1) = sqrt((midPoint(1) - egoPose(1))^2 + (midPoint(2) - egoPose(2))^2);
        d(1,2) = egoSpeed;
        d(1,3) = d(1,1)/d(1,2);     %add ego TOA
        d(1,4) = 4; % 4 is the location of the ego vehicle itself
        
        % if d(1,1) <= 3
        %     ToAThreshold = 2;
        % else
        %     ToAThreshold = 6;
        % end

        if d(1,1) <= flag
            egoEnter = 1;
        end

    
        % loop through signs (vectorized)
        % if smallest dist 
        % d(:,3) -> TOA = v/dist
    
        if numCars > 0
            for k = 1:numCars
                d(k+1,1) = sqrt((midpoint_ego(2)-objectTracks(3,k))^2+(midpoint_ego(1)-objectTracks(1,k))^2); %sqrt((midpoint(1) - (-ObjTracks(3,k)+egoPose(1)))^2 + (midpoint(2) - (ObjTracks(1,k)+egoPose(2)))^2); 
                d(k+1,2) = sqrt((Vmd(1) - objectTracks(2,k))^2 + (Vmd(2) - objectTracks(4,k))^2);
                d(k+1,3) = d(k+1,1)/d(k+1,2); % TOA of other cars
                Objang(k) = atan2d(objectTracks(1,k), -objectTracks(3,k));
                                
                % Identify cars location (direction) wrt ego
                if Objang(k) <= 60
                    d(k+1,4) = 1; % 1 = E, 2 = N, 3 = W
                elseif Objang(k) > 60  && Objang(k) < 120
                    d(k+1,4) = 2; % 1 = E, 2 = N, 3 = W
                elseif Objang(k) >= 120
                    d(k+1,4) = 3; % 1 = E, 2 = N, 3 = W
                end

                % Identifying leaving cars
                
                % ActorHeading = atan2d(ObjTracks(2,k) - Vmd(1), -ObjTracks(4,k) - Vmd(2));
                ActorHeading(k) = atan2d(objectTracks(2,k), objectTracks(4,k));
                actorExitTheta = ActorHeading(k) - atan2d(midpoint_ego(1)-objectTracks(1,k),midpoint_ego(2)-objectTracks(3,k));
                if actorExitTheta > 180
                    actorExitang(k) = actorExitTheta - 360;
                elseif actorExitTheta < -180
                    actorExitang(k) = actorExitTheta + 360;
                else
                    actorExitang(k) = actorExitTheta;
                end
                %actorExitdist = sqrt((midpoint_ego(2)-ObjTracks(3,k))^2+(midpoint_ego(1)-ObjTracks(1,k))^2);
                

                if abs(actorExitang(k)) >= 135 && d(k+1,1) >= 10 
                    d(k+1,5) = 1; % left the ints
                else
                    d(k+1,5) = 0; % did not leave
                end

    
            end
    
            if numSS == 4 
                % Assign priorities based on rank TOA #1, before vehicle stops
                % d1 = d(d(:,1)~=0,:);
                [car, SSPriority] = sort(d(d(:,1)~=0 & d(:,5)==0));
                % priorityTable(:, 1:2) = [car, priority];
        
                tempPriority = find(SSPriority == 1); % ego SS priority
                if ~isempty(tempPriority)
                    egoSSPriority = tempPriority(1);
                end
            
            elseif numSS >= 1 && numSS < 4
                [car, SSPriority] = sort(d((d(:,4)==2 | d(:,4)==4) & d(:,5)==0));
                tempPriority = find(SSPriority == 1); % ego SS priority
                if ~isempty(tempPriority)
                    egoSSPriority = tempPriority(1);              
                end
                ToAClearance = double(all(d(d(:,1)~=0 & d(:,5)==0 & d(:,4)~=4,3) > ToAThreshold));
                
            end
    
        end
    end
    
    
    if ToAClearance == 1 && egoSSPriority == 1 && egoEnter == 1
        process = 0;
    else
        process = 1;
    end
    
    % if egoSpeed <= VelStop
    %     if SSPriority ~= 1
    %         % for all vehicles with higher priority
    %         % provide indicator signals to identify conflicts
    %         % check indicator signs/conflicts and update priority based on that
    %         % code to define leavingScene for other vehicles:
    %         % update priority table
    % 
    %     end
    % end
    
    
    
    

% elseif egoExit == 0
    

end
